simulink subsystem "MFTiresMultibodySSC"  (R2023b)
settings: Solver=VariableStepAuto  StartTime=0.0  StopTime=10.0  RelTol=1e-3
undefined symbols (not defined in the file): AxlFL, AxlFR, AxlRL, AxlRR, PlntVehMultiBody, WheelFL, WheelFR, WheelRL, WheelRR, X, Y, Z
libraries: sm_lib x68, nesl_utility x52, fl_lib x8
(part 4 of 4)

== system MFTiresMultibodySSC/Bus Creation/Omega ==
  Info : Inport
  Bus Selector : BusSelector  OutputSignals=FL.Omega,FR.Omega,RL.Omega,RR.Omega
  Vector Concatenate : Concatenate  NumInputs=4
  Omega : Outport  VectorParamsAs1DForOutWhenUnconnected=off
  wires:
  Bus Selector/2 -> Vector Concatenate/2  "<Omega>"
  Bus Selector/4 -> Vector Concatenate/4  "<Omega>"
  Bus Selector/1 -> Vector Concatenate/1  "<Omega>"
  Bus Selector/3 -> Vector Concatenate/3  "<Omega>"
  Vector Concatenate/1 -> Omega/1
  Info/1 -> Bus Selector/1

== system MFTiresMultibodySSC/Bus Creation/Re ==
  Info : Inport
  Bus Selector : BusSelector  OutputSignals=FL.Re,FR.Re,RL.Re,RR.Re
  Vector Concatenate : Concatenate  NumInputs=4
  Re : Outport  VectorParamsAs1DForOutWhenUnconnected=off
  wires:
  Bus Selector/3 -> Vector Concatenate/3  "<Re>"
  Bus Selector/4 -> Vector Concatenate/4  "<Re>"
  Vector Concatenate/1 -> Re/1
  Info/1 -> Bus Selector/1
  Bus Selector/2 -> Vector Concatenate/2  "<Re>"
  Bus Selector/1 -> Vector Concatenate/1  "<Re>"

== system MFTiresMultibodySSC/Bus Creation/z ==
  Constant{,1..3} (4 alike) : Constant  Value=0  SampleTime=-1
  Vector Concatenate : Concatenate  NumInputs=4
  Out1 : Outport  VectorParamsAs1DForOutWhenUnconnected=off
  wires:
  Vector Concatenate/1 -> Out1/1
  Constant/1 -> Vector Concatenate/1  "z"
  Constant1/1 -> Vector Concatenate/2  "z"
  Constant2/1 -> Vector Concatenate/3  "z"
  Constant3/1 -> Vector Concatenate/4  "z"

== system MFTiresMultibodySSC/Bus Creation/zdot ==
  Constant{,1..3} (4 alike) : Constant  Value=0  SampleTime=-1
  Vector Concatenate : Concatenate  NumInputs=4
  Out1 : Outport  VectorParamsAs1DForOutWhenUnconnected=off
  wires:
  Constant3/1 -> Vector Concatenate/4  "zdot"
  Constant2/1 -> Vector Concatenate/3  "zdot"
  Constant1/1 -> Vector Concatenate/2  "zdot"
  Constant/1 -> Vector Concatenate/1  "zdot"
  Vector Concatenate/1 -> Out1/1
